simulink model "CONT_PID_IZAJE"  (R2024b)
settings: Solver=VariableStepAuto  StartTime=0.0  StopTime=10.0  RelTol=1e-3
undefined symbols (not defined in the file): b_eqh, ih, J_eqh, n_h, rhd, T_s2, w_pos_h
settings Model: Creator=juani  LastModifiedBy=juani

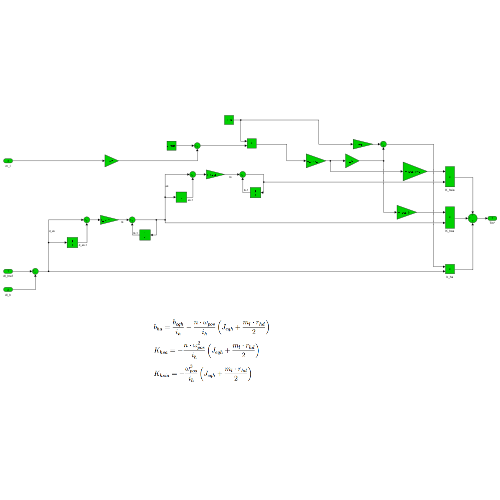
[thumbnail: Simulink's stored preview of the top-level diagram]
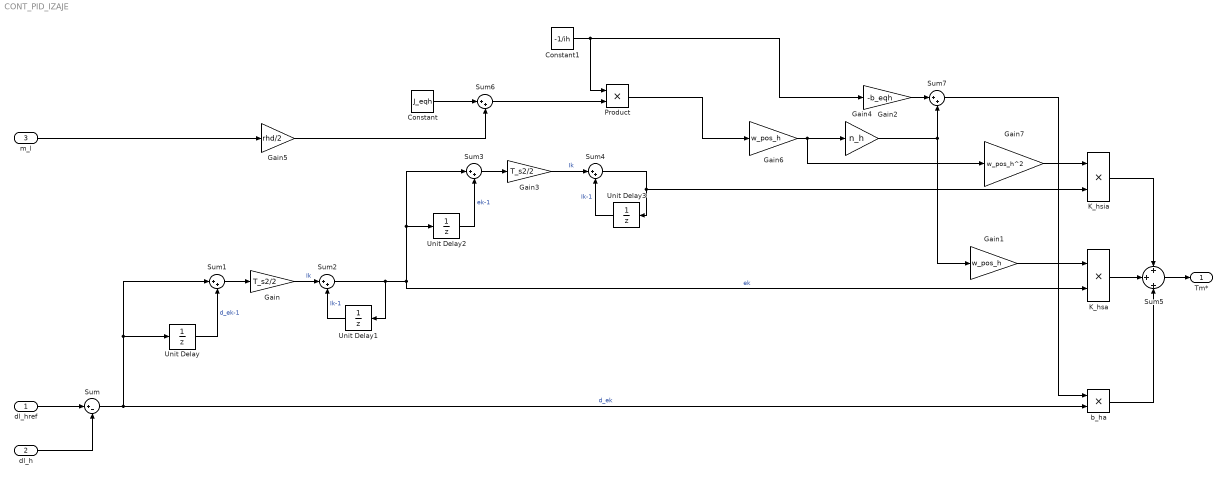
== system CONT_PID_IZAJE ==
  dl_href : Inport
  dl_h : Inport  Port=2
  m_l : Inport  Port=3
  Constant : Constant  Value=J_eqh
  Constant1 : Constant  Value=-1/ih
  Gain : Gain  Gain=T_s2/2
  Gain1 : Gain  Gain=w_pos_h
  Gain2 : Gain  Gain=-b_eqh
  Gain3 : Gain  Gain=T_s2/2
  Gain4 : Gain  Gain=n_h
  Gain5 : Gain  Gain=rhd/2
  Gain6 : Gain  Gain=w_pos_h
  Gain7 : Gain  Gain=w_pos_h^2
  K_hsa : Product
  K_hsia : Product
  Product : Product
  Sum : Sum  Inputs=|+-
  Sum{1..4,6..7} (6 alike) : Sum  Inputs=|++
  Sum5 : Sum  Inputs=+|+|+
  Unit Delay{,1..3} (4 alike) : UnitDelay  SampleTime=-1  HasFrameUpgradeWarning=on
  b_ha : Product
  Tm* : Outport
  wires:
  dl_h/1 -> Sum/2
  dl_href/1 -> Sum/1
  Sum/1 -> b_ha/2, Unit Delay/1, Sum1/1  "d_ek"
  Unit Delay/1 -> Sum1/2  "d_ek-1"
  Sum1/1 -> Gain/1
  Gain/1 -> Sum2/1  "Ik"
  Unit Delay1/1 -> Sum2/2  "Ik-1"
  Sum2/1 -> Unit Delay1/1, Sum3/1, Unit Delay2/1, K_hsa/2  "ek"
  Sum3/1 -> Gain3/1
  Unit Delay2/1 -> Sum3/2  "ek-1"
  Sum4/1 -> Unit Delay3/1, K_hsia/2
  Unit Delay3/1 -> Sum4/2  "Ik-1"
  Gain3/1 -> Sum4/1  "Ik"
  K_hsia/1 -> Sum5/1
  K_hsa/1 -> Sum5/2
  b_ha/1 -> Sum5/3
  Sum5/1 -> Tm*/1
  Constant/1 -> Sum6/1
  m_l/1 -> Gain5/1
  Gain5/1 -> Sum6/2
  Product/1 -> Gain6/1
  Gain2/1 -> Sum7/1
  Gain6/1 -> Gain7/1, Gain4/1
  Constant1/1 -> Gain2/1, Product/1
  Sum6/1 -> Product/2
  Sum7/1 -> b_ha/1
  Gain1/1 -> K_hsa/1
  Gain4/1 -> Gain1/1, Sum7/2
  Gain7/1 -> K_hsia/1
